simulink model "Quadcopter_stud2015"  (Simulink 8.5)
settings: Solver=ode3  SolverMode=SingleTasking  StartTime=0.0  StopTime=100  FixedStep=0.001  RelTol=1e-3
undefined symbols (not defined in the file or in its folder): dronemodel, get, hot
libraries: dspnetwork x2, etargetslib x1, mblibv1 x1, vrlib x1, simulink x1, dspsnks4 x1
settings Model: Creator=zigg  LastModifiedBy=zigg  CovMetricSettings=dwe  CovHtmlReporting=off  covSaveCumulativeToWorkspaceVar=off  CovSaveSingleToWorkspaceVar=off  CovExternalEMLEnable=on
settings DataIOCC: LimitDataPoints=off  SaveFormat=Dataset  SignalLoggingSaveFormat=Dataset
settings OptimizationCC: ExpressionDepthLimit=128
settings DebuggingCC: UnderspecifiedInitializationDetection=Simplified  MergeDetectMultiDrivingBlocksExec=error  FcnCallInpInsideContextMsg=EnableAllAsError  StateNameClashWarn=none  SFUnexpectedBacktrackingDiag=error  SFNoUnconditionalDefaultTransitionDiag=error
settings HardwareCC: ProdBitPerPointer=64  ProdLargestAtomicFloat=Float  ProdIntDivRoundTo=Zero  ProdEndianess=LittleEndian  ProdHWDeviceType=Specified
settings ModelReferenceCC: PropagateSignalLabelsOutOfModel=on
settings GRTTargetCC: TargetLangStandard=C99 (ISO)  GeneratePreprocessorConditionals=Use local settings  CombineOutputUpdateFcns=on  GRTInterface=off

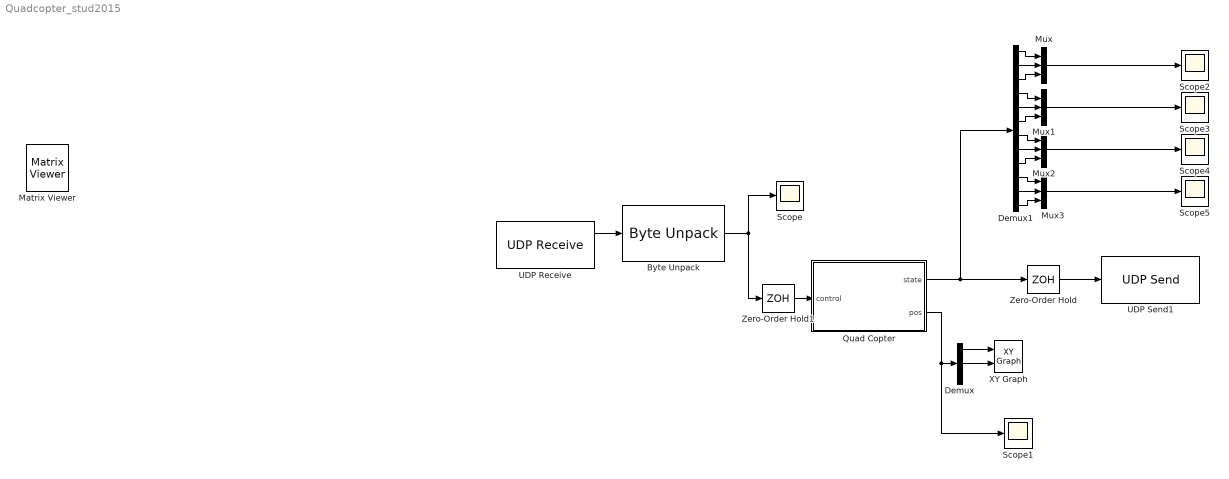
== system Quadcopter_stud2015 ==
  Byte Unpack : etargetslib/Byte Unpack  dimensions={[4]}  datatypes={'double'}  byteAlign=1
  Demux : Demux  Outputs=3
  Demux1 : Demux  Outputs=12
  Mux{,1..3} (4 alike) : Mux  Inputs=3
  Quad Copter : Subsystem
  Scope{,1..5} (6 alike) : Scope
      Scope settings: TimeRange=auto  MaxDataPoints=5000  SaveToWorkspace=off  SaveName=ScopeData  YMin=-0.80889  YMax=1.67512  SampleTime=-1
      Scope1 settings: TimeRange=auto  MaxDataPoints=5000  SaveToWorkspace=off  YMin=-0.03817  YMax=0.28061  SampleTime=-1
      Scope2 settings: TimeRange=auto  MaxDataPoints=5000  SaveToWorkspace=off  SaveName=ScopeData2  YMin=-1.26258  YMax=1.42775  SampleTime=-1
      Scope3 settings: TimeRange=auto  MaxDataPoints=5000  SaveToWorkspace=off  SaveName=ScopeData3  YMin=-41745161341028635266904900723802112.00000  YMax=41835259513013165231493040876552192.00000  SampleTime=-1
      Scope4 settings: TimeRange=auto  MaxDataPoints=5000  SaveToWorkspace=off  SaveName=ScopeData4  YMin=-3.16843  YMax=2.55595  SampleTime=-1
      Scope5 settings: TimeRange=auto  MaxDataPoints=5000  SaveToWorkspace=off  SaveName=ScopeData5  YMin=-124083574141231526363786560705880637043313122335498294732192175333531917753379844375079562440588598769793979956002391202209046263482670404690692647685563687116490440698657686468587348068809090007040.00000  YMax=85815314521898447887506626206619620496955852810638829978215292653564095480350618283421790405146534256292267484009278159868236243760942414968457676421487013622573953345822982855863617888913360683008.00000  SampleTime=-1
  UDP Receive : dspnetwork/UDP Receive  localURL='0.0.0.0'  localPort=4000  remoteURL='192.168.2.239'  remotePort=-1  recvBufferSize=8192  dims=32  signalDatatype=uint8  isVarSize=off  showBlockingTime=off  blockingTime=0  sampletime=0.001  blockPlatform=[]
  UDP Send1 : dspnetwork/UDP Send  remoteURL='192.168.2.239'  remotePort=4000  localURL='0.0.0.0'  localPortSource=Automatically determine  localPort=-1  sampletime=-1  blockPlatform=[]  separateLengthPort=0
  XY Graph : simulink/Sinks/XY Graph  xmin=-2  xmax=2  ymin=-2  ymax=2  st=-1
  Zero-Order Hold : ZeroOrderHold  SampleTime=0.001
  Zero-Order Hold1 : ZeroOrderHold  SampleTime=0.001
  Matrix Viewer : dspsnks4/Matrix Viewer  IOType=viewer  ImageParams=off  CMapStr=hot(256)  AxisColorbar=on  AxisParams=off  AxisOrigin=Upper left corner  XLabel=X-axis  YLabel=Y-axis  ZLabel=Z-axis  FigPos=get(0,'defaultfigureposition')  AxisZoom=off
      settings: YMin=-1.0  YMax=1.0
  wires:
  UDP Receive/1 -> Byte Unpack/1
  Byte Unpack/1 -> Zero-Order Hold1/1, Scope/1
  Quad Copter/1(state) -> Demux1/1, Zero-Order Hold/1
  Quad Copter/2(pos) -> Scope1/1, Demux/1
  Demux/1 -> XY Graph/1
  Demux/2 -> XY Graph/2
  Demux1/1 -> Mux/1
  Demux1/2 -> Mux/2
  Demux1/3 -> Mux/3
  Mux/1 -> Scope2/1
  Mux1/1 -> Scope3/1
  Demux1/4 -> Mux1/1
  Demux1/5 -> Mux1/2
  Demux1/6 -> Mux1/3
  Mux2/1 -> Scope4/1
  Demux1/7 -> Mux2/1
  Demux1/8 -> Mux2/2
  Demux1/9 -> Mux2/3
  Mux3/1 -> Scope5/1
  Demux1/12 -> Mux3/3
  Demux1/11 -> Mux3/2
  Demux1/10 -> Mux3/1
  Zero-Order Hold/1 -> UDP Send1/1
  Zero-Order Hold1/1 -> Quad Copter/1(control)

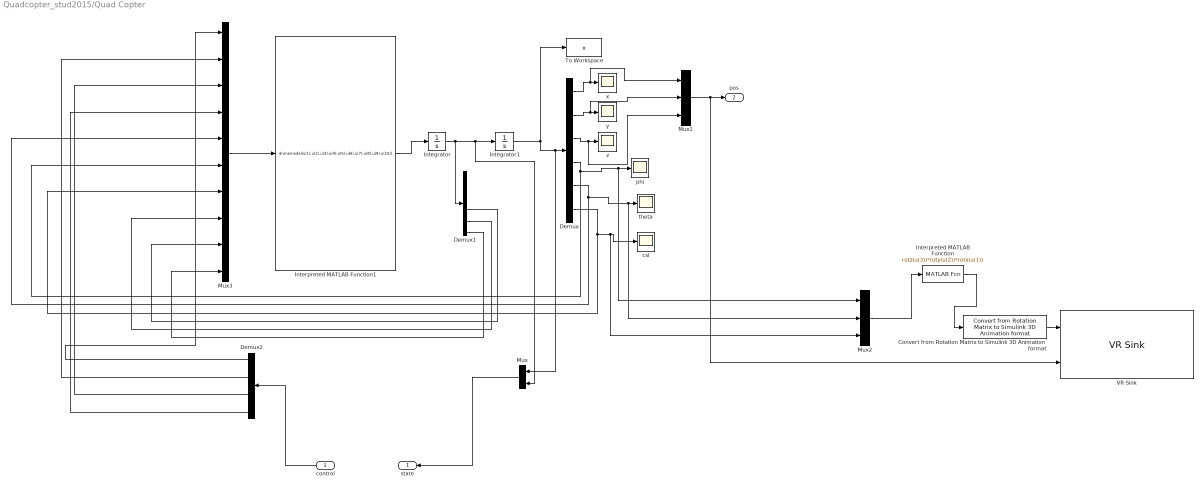
== system Quadcopter_stud2015/Quad Copter ==
  control : Inport  PortDimensions=4
  Convert from Rotation Matrix to Simulink 3D Animation format : mblibv1/Utilities/Convert from Rotation Matrix to Simulink 3D Animation format
  Demux : Demux  Outputs=6
  Demux1 : Demux  Outputs=6
  Demux2 : Demux
  Integrator : Integrator
  Integrator1 : Integrator
  Interpreted MATLAB Function : MATLABFcn  MATLABFcn=rotz(u(3))*roty(u(2))*rotx(u(1))  OutputDimensions=9
  Interpreted MATLAB Function1 : MATLABFcn  MATLABFcn=dronemodel(u(1),u(2),u(3),u(4),u(5),u(6),u(7),u(8),u(9),u(10))  Output1D=off
  Mux : Mux  Inputs=2
      settings: DisplayOption=signals
  Mux1 : Mux  Inputs=3
  Mux2 : Mux  Inputs=3
  Mux3 : Mux  Inputs=10
  To Workspace : ToWorkspace  VariableName=x  SampleTime=-1
  VR Sink : vrlib/VR Sink  InstantiateOnLoad=on  SampleTime=0.1  ViewEnable=on  RemoteChange=off  RemoteView=off  FieldsWritten=Drone.rotation.4.1.1.double#Drone.translation.3.1.1.double  WorldFileName=drone.wrl  AutoView=off  VideoDimensions=[]  AllowVariableSize=off
  csi : Scope
      settings: TimeRange=auto  MaxDataPoints=5000  SaveToWorkspace=off  SaveName=ScopeData5  YMin=-1.17153  YMax=1.17039  SampleTime=-1
  phi : Scope
      settings: TimeRange=auto  MaxDataPoints=5000  SaveToWorkspace=off  SaveName=ScopeData3  YMin=-0.04291  YMax=0.05573  SampleTime=-1
  theta : Scope
      settings: TimeRange=auto  MaxDataPoints=5000  SaveToWorkspace=off  SaveName=ScopeData4  YMin=-0.03736  YMax=0.02141  SampleTime=-1
  x : Scope
      settings: TimeRange=auto  MaxDataPoints=5000  SaveToWorkspace=off  SaveName=ScopeData  YMin=-1.23873  YMax=1.23815  SampleTime=-1
  y : Scope
      settings: TimeRange=auto  MaxDataPoints=5000  SaveToWorkspace=off  YMin=-1.2418  YMax=1.24065  SampleTime=-1
  z : Scope
      settings: TimeRange=auto  MaxDataPoints=5000  SaveToWorkspace=off  SaveName=ScopeData2  YMin=0.13098  YMax=1.23069  SampleTime=-1
  state : Outport
  pos : Outport  Port=2
  wires:
  Integrator/1 -> Demux1/1, Mux/2, Integrator1/1
  Interpreted MATLAB Function1/1 -> Integrator/1
  Integrator1/1 -> Mux/1, Demux/1, To Workspace/1
  Demux/1 -> Mux1/1, x/1
  Demux/2 -> Mux1/2, y/1
  Demux/3 -> Mux1/3, z/1
  Demux1/4 -> Mux3/9
  Demux1/5 -> Mux3/8
  Demux1/6 -> Mux3/10
  Mux/1 -> state/1
  Demux2/1 -> Mux3/1
  Demux2/2 -> Mux3/2
  Demux2/3 -> Mux3/3
  Demux2/4 -> Mux3/4
  control/1 -> Demux2/1
  Mux2/1 -> Interpreted MATLAB Function/1
  Convert from Rotation Matrix to Simulink 3D Animation format/1 -> VR Sink/1
  Demux/5 -> Mux3/5, Mux2/2, theta/1
  Demux/6 -> Mux3/7, Mux2/3, csi/1
  Demux/4 -> Mux3/6, Mux2/1, phi/1
  Interpreted MATLAB Function/1 -> Convert from Rotation Matrix to Simulink 3D Animation format/1
  Mux1/1 -> VR Sink/2, pos/1
  Mux3/1 -> Interpreted MATLAB Function1/1
